simulink model "ctrl_typeA"  (R2016b)
settings: Solver=ode45  StartTime=0.0  StopTime=12.0  RelTol=1e-3  EnableMultiTasking=on
undefined symbols (not defined in the file): cMat_BF, cMat_IM, cMat_MN, cMat_TM, gain_actBFGAS, gain_actBFL, gain_actBFP, gain_actBFR, gain_actBFT, gain_actBFV, gain_actBFY, gain_actF0GAS, gain_actF1GAS, gain_actF2GAS, gain_actF3GAS, gain_actIML, gain_actIMP, gain_actIMR, gain_actIMT, gain_actIMV, gain_actIMY, gain_actIPL, gain_actIPT, gain_actIPY, gain_actMNL, gain_actMNP, gain_actMNR, gain_actMNT, gain_actMNV, gain_actMNY, gain_actTML, gain_actTMP, gain_actTMY, gainBFGAS, gainBFL, gainBFP, gainBFR, gainBFT, gainBFV, gainBFY, gainF0GAS, gainF1GAS, gainF2GAS, gainF3GAS, gainHieBFP, gainHieBFR, gainHieBFY, gainHieIML, gainHieIMP, gainHieIMY, gainHieIPL, gainHieIPY, gainHieMNL, gainHieMNP, gainHieMNY, gainIML, gainIMP, gainIMR, gainIMT, gainIMV ... (+24)
libraries: cstblocks x54
(part 2 of 2)

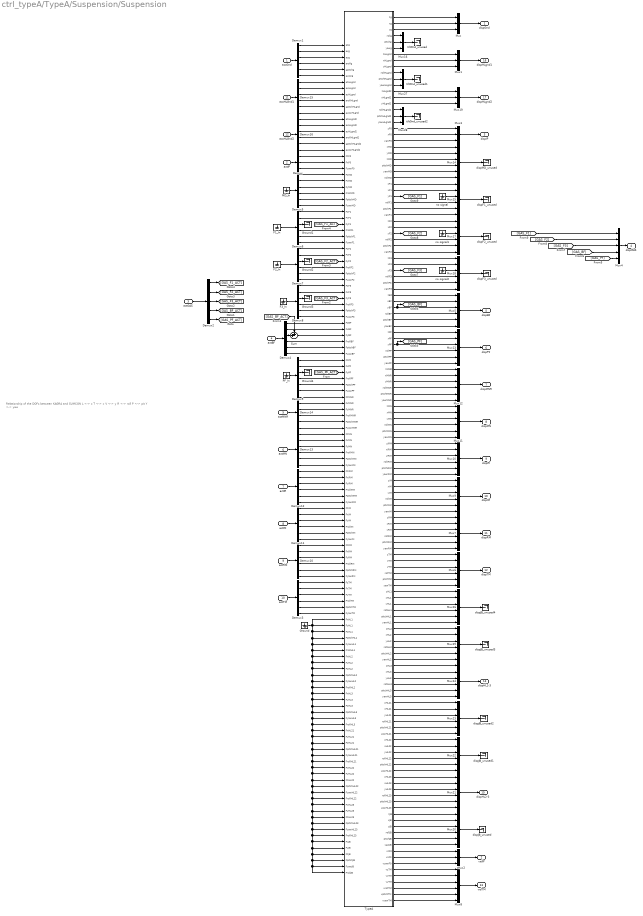
== system ctrl_typeA/TypeA/Suspension/Suspension ==
  note: Relationship of the DOFs
      | between KAGRA and SUMCON
      |
      | L <-> z
      | T <-> x
      | V <-> y
      | R <-> roll
      | P <-> pit
      | Y <-> yaw
  accGnd : Inport
  actIP : Inport  Port=2
  actGAS : Inport  Port=3
  actBF : Inport  Port=4
  actMNR : Inport  Port=5
  actMN : Inport  Port=6
  actIR : Inport  Port=7
  actIM : Inport  Port=8
  actRM : Inport  Port=9
  actTM : Inport  Port=10
  accHLGnd1 : Inport  Port=11
  accHLGnd2 : Inport  Port=12
  Demux : Demux  Outputs=3
  Demux{1,3..16} (15 alike) : Demux  Outputs=6
  Demux2 : Demux  Outputs=5
  F1_In : Ground
  F2_In : Ground
  F3_In : Ground
  Ground : Ground
  Ground{1..4} (4 alike) : Terminator
  MD_In : Ground
  Mux{,1..3,16,19,27..28} (8 alike) : Mux  Inputs=3
  Mux{5..15,17..18,20..26} (20 alike) : Mux  Inputs=6
  Mux4 : Mux  Inputs=5
  PF_In : Ground
  Sum : Sum  Inputs=++|
  TypeA : Subsystem
  dispF1_unused : Terminator
  dispF2_unused : Terminator
  dispF3_unused : Terminator
  dispJB_unused{,1..4} (5 alike) : Terminator
  dispMD_unused : Terminator
  no signal : Ground
  no signal1 : Ground
  no signal2 : Ground
  tiltGnd_unused : Terminator
  tiltGnd_unused1 : Terminator
  tiltGnd_unused2 : Terminator
  dispGnd : Outport
  velIP : Outport  Port=2
  dispIP : Outport  Port=3
  dispGAS : Outport  Port=4
  dispBF : Outport  Port=5
  dispPF : Outport  Port=6
  dispMNR : Outport  Port=7
  dispMN : Outport  Port=8
  dispIR : Outport  Port=9
  dispIM : Outport  Port=10
  dispRM : Outport  Port=11
  dispTM : Outport  Port=12
  velTM : Outport  Port=13
  dispHL1-3 : Outport  Port=14
  dispHL2-3 : Outport  Port=15
  dispHLgnd1 : Outport  Port=16
  dispHLgnd2 : Outport  Port=17
  wires:
  Mux/1 -> dispGnd/1
  Mux2/1 -> velIP/1
  Mux3/1 -> dispIP/1
  Mux4/1 -> dispGAS/1
  Mux5/1 -> dispBF/1
  Mux6/1 -> dispTM/1
  actIP/1 -> Demux/1
  accGnd/1 -> Demux1/1
  actTM/1 -> Demux3/1
  Demux4/3 -> Sum/2
  actBF/1 -> Demux4/1
  actGAS/1 -> Demux2/1
  MD_In/1 -> Demux5/1
  F1_In/1 -> Demux6/1
  F2_In/1 -> Demux7/1
  F3_In/1 -> Demux8/1
  Demux4/1 -> TypeA/46(FzBF)
  PF_In/1 -> Demux9/1
  actRM/1 -> Demux10/1
  actIM/1 -> Demux11/1
  actIR/1 -> Demux12/1
  actMN/1 -> Demux13/1
  actMNR/1 -> Demux14/1
  Demux10/5 -> TypeA/86(FpitchRM)
  Demux10/4 -> TypeA/85(FrollRM)
  Demux10/3 -> TypeA/84(FyRM)
  Demux10/1 -> TypeA/82(FzRM)
  Demux10/2 -> TypeA/83(FxRM)
  Demux3/3 -> TypeA/90(FyTM)
  Demux3/1 -> TypeA/88(FzTM)
  Demux3/2 -> TypeA/89(FxTM)
  Demux3/4 -> TypeA/91(FrollTM)
  Demux3/5 -> TypeA/92(FpitchTM)
  Demux3/6 -> TypeA/93(FyawTM)
  Mux7/1 -> dispRM/1
  Mux8/1 -> velTM/1
  Mux9/1 -> dispIM/1
  Mux10/1 -> dispIR/1
  Mux11/1 -> dispMN/1
  Mux12/1 -> dispMNR/1
  Mux13/1 -> dispPF/1
  Mux14/1 -> dispMD_unused/1
  Mux15/1 -> dispF1_unused/1
  Mux16/1 -> tiltGnd_unused/1
  Mux17/1 -> dispF2_unused/1
  Mux18/1 -> dispF3_unused/1
  TypeA/2(xg) -> Mux/2
  TypeA/1(zg) -> Mux/1
  TypeA/138(vyawF0) -> Mux2/3
  TypeA/20(xF0) -> Mux3/2
  TypeA/19(zF0) -> Mux3/1
  TypeA/21(yawF0) -> Mux3/3
  TypeA/24(zMD) -> Mux14/3
  TypeA/25(pitchMD) -> Mux14/4
  TypeA/26(yawMD) -> Mux14/5
  TypeA/27(rollMD) -> Mux14/6
  TypeA/48(yBF) -> Mux5/3, [GAS_BF]
  TypeA/54(yPF) -> [GAS_PF], Mux13/3
  TypeA/28(zF1) -> Mux15/1
  TypeA/29(xF1) -> Mux15/2
  TypeA/33(yawF1) -> Mux15/6
  TypeA/31(rollF1) -> Mux15/4
  TypeA/32(pitchF1) -> Mux15/5
  TypeA/34(zF2) -> Mux17/1
  TypeA/35(xF2) -> Mux17/2
  TypeA/37(rollF2) -> Mux17/4
  TypeA/39(yawF2) -> Mux17/6
  TypeA/38(pitchF2) -> Mux17/5
  TypeA/40(zF3) -> Mux18/1
  TypeA/41(xF3) -> Mux18/2
  TypeA/45(yawF3) -> Mux18/6
  TypeA/44(pitchF3) -> Mux18/5
  TypeA/43(rollF3) -> Mux18/4
  TypeA/50(pitchBF) -> Mux5/5
  TypeA/51(yawBF) -> Mux5/6
  TypeA/49(rollBF) -> Mux5/4
  TypeA/47(xBF) -> Mux5/2
  TypeA/46(zBF) -> Mux5/1
  TypeA/57(yawPF) -> Mux13/6
  TypeA/52(zPF) -> Mux13/1
  TypeA/53(xPF) -> Mux13/2
  TypeA/55(rollPF) -> Mux13/4
  TypeA/56(pitchPF) -> Mux13/5
  TypeA/59(xMNR) -> Mux12/2
  TypeA/63(yawMNR) -> Mux12/6
  TypeA/60(yMNR) -> Mux12/3
  TypeA/61(rollMNR) -> Mux12/4
  TypeA/58(zMNR) -> Mux12/1
  TypeA/62(pitchMNR) -> Mux12/5
  TypeA/67(rollMN) -> Mux11/4
  TypeA/64(zMN) -> Mux11/1
  TypeA/66(yMN) -> Mux11/3
  TypeA/65(xMN) -> Mux11/2
  TypeA/69(yawMN) -> Mux11/6
  TypeA/68(pitchMN) -> Mux11/5
  TypeA/74(pitchIRM) -> Mux10/5
  TypeA/72(yIRM) -> Mux10/3
  TypeA/75(yawIRM) -> Mux10/6
  TypeA/73(rollIRM) -> Mux10/4
  TypeA/71(xIRM) -> Mux10/2
  TypeA/70(zIRM) -> Mux10/1
  TypeA/76(zIM) -> Mux9/1
  TypeA/78(yIM) -> Mux9/3
  TypeA/77(xIM) -> Mux9/2
  TypeA/139(vzTM) -> Mux8/1
  TypeA/140(vxTM) -> Mux8/2
  TypeA/141(vyTM) -> Mux8/3
  TypeA/88(zTM) -> Mux6/1
  TypeA/89(xTM) -> Mux6/2
  TypeA/90(yTM) -> Mux6/3
  TypeA/82(zRM) -> Mux7/1
  TypeA/83(xRM) -> Mux7/2
  TypeA/84(yRM) -> Mux7/3
  TypeA/79(rollIM) -> Mux9/4
  TypeA/80(pitchIM) -> Mux9/5
  TypeA/81(yawIM) -> Mux9/6
  TypeA/85(rollRM) -> Mux7/4
  TypeA/86(pitchRM) -> Mux7/5
  TypeA/87(yawRM) -> Mux7/6
  TypeA/91(rollTM) -> Mux6/4
  TypeA/92(pitchTM) -> Mux6/5
  TypeA/93(yawTM) -> Mux6/6
  TypeA/22(xMD) -> Mux14/1
  TypeA/23(yMD) -> Mux14/2
  TypeA/137(vxF0) -> Mux2/2
  TypeA/136(vzF0) -> Mux2/1
  TypeA/3(yg) -> Mux/3
  Demux10/6 -> TypeA/87(FyawRM)
  Demux11/1 -> TypeA/76(FzIM)
  Demux11/2 -> TypeA/77(FxIM)
  Demux11/3 -> TypeA/78(FyIM)
  Demux11/4 -> TypeA/79(FrollIM)
  Demux11/5 -> TypeA/80(FpitchIM)
  Demux11/6 -> TypeA/81(FyawIM)
  Demux12/1 -> TypeA/70(FzIRM)
  Demux12/2 -> TypeA/71(FxIRM)
  Demux12/3 -> TypeA/72(FyIRM)
  Demux12/4 -> TypeA/73(FrollIRM)
  Demux12/5 -> TypeA/74(FpitchIRM)
  Demux12/6 -> TypeA/75(FyawIRM)
  Demux13/1 -> TypeA/64(FzMN)
  Demux13/2 -> TypeA/65(FxMN)
  Demux13/3 -> TypeA/66(FyMN)
  Demux13/4 -> TypeA/67(FrollMN)
  Demux13/5 -> TypeA/68(FpitchMN)
  Demux13/6 -> TypeA/69(FyawMN)
  Demux14/1 -> TypeA/58(FzMNR)
  Demux14/2 -> TypeA/59(FxMNR)
  Demux14/3 -> TypeA/60(FyMNR)
  Demux14/4 -> TypeA/61(FrollMNR)
  Demux14/5 -> TypeA/62(FpitchMNR)
  Demux14/6 -> TypeA/63(FyawMNR)
  Demux9/1 -> TypeA/52(FzPF)
  Demux9/2 -> TypeA/53(FxPF)
  Demux4/2 -> TypeA/47(FxBF)
  Sum/1 -> TypeA/48(FyBF)
  Demux4/4 -> TypeA/49(FrollBF)
  Demux4/5 -> TypeA/50(FpitchBF)
  Demux4/6 -> TypeA/51(FyawBF)
  Demux8/1 -> TypeA/40(FzF3)
  Demux8/2 -> TypeA/41(FxF3)
  Demux7/1 -> TypeA/34(FzF2)
  Demux7/2 -> TypeA/35(FxF2)
  Demux6/1 -> TypeA/28(FzF1)
  Demux6/2 -> TypeA/29(FxF1)
  Demux/1 -> TypeA/19(FzF0)
  Demux/2 -> TypeA/20(FxF0)
  Demux/3 -> TypeA/21(FyawF0)
  Demux1/1 -> TypeA/1(azg)
  Demux1/2 -> TypeA/2(axg)
  Demux1/3 -> TypeA/3(ayg)
  Demux1/4 -> TypeA/4(arollg)
  Demux1/5 -> TypeA/5(apitchg)
  Demux1/6 -> TypeA/6(ayawg)
  Mux20/1 -> dispJB_unused/1
  Mux21/1 -> dispHL2-3/1
  Mux22/1 -> dispJB_unused1/1
  Mux23/1 -> dispJB_unused2/1
  Mux24/1 -> dispHL1-3/1
  Mux25/1 -> dispJB_unused3/1
  Mux26/1 -> dispJB_unused4/1
  TypeA/7(zHLgnd) -> Mux1/1
  TypeA/8(xHLgnd) -> Mux1/2
  TypeA/9(yHLgnd) -> Mux1/3
  Mux1/1 -> dispHLgnd1/1
  Mux19/1 -> dispHLgnd2/1
  TypeA/15(yHLgnd2) -> Mux19/3
  TypeA/13(zHLgnd2) -> Mux19/1
  TypeA/14(xHLgnd2) -> Mux19/2
  Mux27/1 -> tiltGnd_unused1/1
  Mux28/1 -> tiltGnd_unused2/1
  Ground/1 -> TypeA/96(FzHL1), TypeA/97(FpitchHL1), TypeA/98(FyawHL1), TypeA/99(FrollHL1), TypeA/100(FxHL2), TypeA/101(FyHL2), TypeA/102(FzHL2), TypeA/103(FpitchHL2), TypeA/104(FyawHL2), TypeA/105(FrollHL2), TypeA/106(FxHL3), TypeA/107(FyHL3), TypeA/108(FzHL3), TypeA/109(FpitchHL3), TypeA/110(FyawHL3), TypeA/111(FrollHL3), TypeA/112(FxHL21), TypeA/113(FyHL21), TypeA/114(FzHL21), TypeA/115(FpitchHL21), TypeA/116(FyawHL21), TypeA/117(FrollHL21), TypeA/118(FxHL22), TypeA/119(FyHL22), TypeA/120(FzHL22), TypeA/121(FpitchHL22), TypeA/122(FyawHL22), TypeA/123(FrollHL22), TypeA/124(FxHL23), TypeA/125(FyHL23), TypeA/126(FzHL23), TypeA/127(FpitchHL23), TypeA/128(FyawHL23), TypeA/129(FrollHL23), TypeA/130(FxJB), TypeA/131(FyJB), TypeA/132(FzJB), TypeA/133(FpitchJB), TypeA/134(FyawJB), TypeA/135(FrollJB), TypeA/95(FyHL1), TypeA/94(FxHL1)
  Demux15/4 -> TypeA/10(arollHLgnd)
  Demux15/5 -> TypeA/11(apitchHLgnd)
  Demux15/1 -> TypeA/7(azHLgnd)
  Demux15/2 -> TypeA/8(axHLgnd)
  Demux15/6 -> TypeA/12(ayawHLgnd)
  accHLGnd1/1 -> Demux15/1
  Demux15/3 -> TypeA/9(ayHLgnd)
  Demux16/4 -> TypeA/16(arollHLgnd2)
  Demux16/5 -> TypeA/17(apitchHLgnd2)
  Demux16/1 -> TypeA/13(azHLgnd2)
  Demux16/2 -> TypeA/14(axHLgnd2)
  Demux16/6 -> TypeA/18(ayawHLgnd2)
  accHLGnd2/1 -> Demux16/1
  Demux16/3 -> TypeA/15(ayHLgnd2)
  Demux5/1 -> TypeA/22(FzMD)
  Demux5/2 -> TypeA/23(FxMD)
  Demux5/3 -> TypeA/24(FyMD)
  Demux5/4 -> TypeA/25(FrollMD)
  Demux5/5 -> TypeA/26(FpitchMD)
  Demux5/6 -> TypeA/27(FyawMD)
  Demux2/1 -> [GAS_F1_ACT]
  Demux2/2 -> [GAS_F2_ACT]
  Demux2/3 -> [GAS_F3_ACT]
  Demux2/4 -> [GAS_BF_ACT]
  Demux2/5 -> [GAS_PF_ACT]
  [GAS_F1_ACT] -> TypeA/30(FyF1)
  Demux6/4 -> TypeA/31(FrollF1)
  Demux6/3 -> Ground1/1
  Demux6/5 -> TypeA/32(FpitchF1)
  Demux6/6 -> TypeA/33(FyawF1)
  [GAS_F2_ACT] -> TypeA/36(FyF2)
  Demux7/5 -> TypeA/38(FpitchF2)
  Demux7/6 -> TypeA/39(FyawF2)
  Demux7/3 -> Ground2/1
  Demux7/4 -> TypeA/37(FrollF2)
  [GAS_F3_ACT] -> TypeA/42(FyF3)
  Demux8/3 -> Ground3/1
  Demux8/6 -> TypeA/45(FyawF3)
  Demux8/5 -> TypeA/44(FpitchF3)
  Demux8/4 -> TypeA/43(FrollF3)
  [GAS_BF_ACT] -> Sum/1
  [GAS_PF_ACT] -> TypeA/54(FyPF)
  Demux9/4 -> TypeA/55(FrollPF)
  Demux9/3 -> Ground4/1
  Demux9/5 -> TypeA/56(FpitchPF)
  Demux9/6 -> TypeA/57(FyawPF)
  TypeA/42(yF3) -> [GAS_F3]
  [GAS_PF] -> Mux4/5
  [GAS_BF] -> Mux4/4
  [GAS_F3] -> Mux4/3
  TypeA/36(yF2) -> [GAS_F2]
  TypeA/30(yF1) -> [GAS_F1]
  [GAS_F2] -> Mux4/2
  [GAS_F1] -> Mux4/1
  TypeA/4(rollg) -> Mux16/1
  TypeA/5(pitchg) -> Mux16/2
  TypeA/10(rollHLgnd) -> Mux27/1
  TypeA/11(pitchHLgnd) -> Mux27/2
  TypeA/16(rollHLgnd2) -> Mux28/1
  TypeA/17(pitchHLgnd2) -> Mux28/2
  no signal/1 -> Mux15/3
  no signal1/1 -> Mux17/3
  no signal2/1 -> Mux18/3
  TypeA/96(yHL1) -> Mux26/3
  TypeA/95(xHL1) -> Mux26/2
  TypeA/94(zHL1) -> Mux26/1
  TypeA/99(yawHL1) -> Mux26/6
  TypeA/98(pitchHL1) -> Mux26/5
  TypeA/97(rollHL1) -> Mux26/4
  TypeA/100(zHL2) -> Mux25/1
  TypeA/101(xHL2) -> Mux25/2
  TypeA/102(yHL2) -> Mux25/3
  TypeA/103(rollHL2) -> Mux25/4
  TypeA/104(pitchHL2) -> Mux25/5
  TypeA/105(yawHL2) -> Mux25/6
  TypeA/107(xHL3) -> Mux24/2
  TypeA/108(yHL3) -> Mux24/3
  TypeA/109(rollHL3) -> Mux24/4
  TypeA/110(pitchHL3) -> Mux24/5
  TypeA/111(yawHL3) -> Mux24/6
  TypeA/106(zHL3) -> Mux24/1
  TypeA/112(zHL21) -> Mux23/1
  TypeA/113(xHL21) -> Mux23/2
  TypeA/114(yHL21) -> Mux23/3
  TypeA/115(rollHL21) -> Mux23/4
  TypeA/116(pitchHL21) -> Mux23/5
  TypeA/117(yawHL21) -> Mux23/6
  TypeA/119(xHL22) -> Mux22/2
  TypeA/120(yHL22) -> Mux22/3
  TypeA/118(zHL22) -> Mux22/1
  TypeA/122(pitchHL22) -> Mux22/5
  TypeA/123(yawHL22) -> Mux22/6
  TypeA/121(rollHL22) -> Mux22/4
  TypeA/125(xHL23) -> Mux21/2
  TypeA/126(yHL23) -> Mux21/3
  TypeA/124(zHL23) -> Mux21/1
  TypeA/128(pitchHL23) -> Mux21/5
  TypeA/129(yawHL23) -> Mux21/6
  TypeA/127(rollHL23) -> Mux21/4
  TypeA/131(xJB) -> Mux20/2
  TypeA/132(yJB) -> Mux20/3
  TypeA/130(zJB) -> Mux20/1
  TypeA/134(pitchJB) -> Mux20/5
  TypeA/135(yawJB) -> Mux20/6
  TypeA/133(rollJB) -> Mux20/4
  TypeA/143(vpitchTM) -> Mux8/5
  TypeA/144(vyawTM) -> Mux8/6
  TypeA/142(vrollTM) -> Mux8/4
  TypeA/6(yawg) -> Mux16/3
  TypeA/12(yawHLgnd) -> Mux27/3
  TypeA/18(yawHLgnd2) -> Mux28/3

== system ctrl_typeA/TypeA/Suspension/aMatrix_BF ==
  aMat_in : Inport
  cMat_BF : Constant  Value=cMat_BF  VectorParams1D=off
  coupling_BF : Product  Multiplication=Matrix(*)
  actBF : Outport
  wires:
  coupling_BF/1 -> actBF/1
  aMat_in/1 -> coupling_BF/2
  cMat_BF/1 -> coupling_BF/1

== system ctrl_typeA/TypeA/Suspension/aMatrix_GAS ==
  aMat_in : Inport
  Add{1..4} (4 alike) : Sum  Inputs=+-
  Demux4 : Demux  Outputs=5
  Mux3 : Mux  Inputs=5
  actGAS : Outport
  wires:
  aMat_in/1 -> Demux4/1
  Mux3/1 -> actGAS/1
  Add1/1 -> Mux3/1
  Add2/1 -> Mux3/2
  Demux4/3 -> Add3/1, Add2/2
  Demux4/2 -> Add1/2, Add2/1
  Demux4/1 -> Add1/1
  Demux4/5 -> Mux3/5, Add4/2
  Add4/1 -> Mux3/4
  Add3/1 -> Mux3/3
  Demux4/4 -> Add3/2, Add4/1

== system ctrl_typeA/TypeA/Suspension/aMatrix_IM ==
  aMat_in : Inport
  Gain : Gain  Gain=-1
  cMat_IM : Constant  Value=cMat_IM  VectorParams1D=off
  coupling_IM : Product  Multiplication=Matrix(*)
  actIR : Outport
  actIM : Outport  Port=2
  wires:
  coupling_IM/1 -> actIM/1, Gain/1
  aMat_in/1 -> coupling_IM/2
  cMat_IM/1 -> coupling_IM/1
  Gain/1 -> actIR/1

== system ctrl_typeA/TypeA/Suspension/aMatrix_MN ==
  aMat_in : Inport
  Gain : Gain  Gain=-1
  cMat_MN : Constant  Value=cMat_MN  VectorParams1D=off
  coupling_MN : Product  Multiplication=Matrix(*)
  actMNR : Outport
  actMN : Outport  Port=2
  wires:
  coupling_MN/1 -> actMN/1, Gain/1
  aMat_in/1 -> coupling_MN/2
  cMat_MN/1 -> coupling_MN/1
  Gain/1 -> actMNR/1

== system ctrl_typeA/TypeA/Suspension/aMatrix_TM ==
  aMat_in : Inport
  Demux : Demux  Outputs=3
  Demux1 : Demux  Outputs=3
  Gain : Gain  Gain=-1
  Ground{,1..5} (6 alike) : Ground
  Mux : Mux  Inputs=6
  Mux1 : Mux  Inputs=6
  cMat_TM : Constant  Value=cMat_TM  VectorParams1D=off
  coupling_TM : Product  Multiplication=Matrix(*)
  actRM : Outport
  actTM : Outport  Port=2
  wires:
  coupling_TM/1 -> Demux1/1, Gain/1
  aMat_in/1 -> coupling_TM/2  "3DoF"
  cMat_TM/1 -> coupling_TM/1
  Gain/1 -> Demux/1
  Demux/1 -> Mux/1
  Demux/2 -> Mux/5
  Demux/3 -> Mux/6
  Demux1/1 -> Mux1/1
  Demux1/3 -> Mux1/6
  Demux1/2 -> Mux1/5
  Ground/1 -> Mux/2
  Ground1/1 -> Mux/3
  Ground2/1 -> Mux/4
  Ground4/1 -> Mux1/3
  Ground3/1 -> Mux1/2
  Ground5/1 -> Mux1/4
  Mux/1 -> actRM/1  "6DoF"
  Mux1/1 -> actTM/1  "6DoF"

== system ctrl_typeA/TypeA/Suspension/sMatrix_BF_LVDT ==
  dispGnd : Inport
  dispBF : Inport  Port=2
  Add2 : Sum  Inputs=-+
  Demux : Demux  Outputs=3
  Ground : Ground
  Ground1 : Ground
  Ground2 : Ground
  Mux : Mux  Inputs=6
  BF_LVDT : Outport
  wires:
  Add2/1 -> BF_LVDT/1  "6DoF"
  dispBF/1 -> Add2/2  "6DoF"
  dispGnd/1 -> Demux/1  "3DoF"
  Demux/1 -> Mux/1  "L"
  Demux/2 -> Mux/2  "T"
  Demux/3 -> Mux/3  "V"
  Ground/1 -> Mux/4  "R"
  Ground1/1 -> Mux/5  "P"
  Mux/1 -> Add2/1
  Ground2/1 -> Mux/6  "Y"

== system ctrl_typeA/TypeA/Suspension/sMatrix_GAS_LVDT ==
  dispGAS : Inport
  dispGND : Inport  Port=2
  Add{1..5} (5 alike) : Sum  Inputs=-+
  Demux : Demux  Outputs=3
  Demux4 : Demux  Outputs=5
  Mux3 : Mux  Inputs=5
  Terminator1 : Terminator
  Terminator2 : Terminator
  GAS_LVDT : Outport
  wires:
  dispGAS/1 -> Demux4/1
  Demux4/1 -> Add2/2, Add1/1  "VF1"
  Demux4/2 -> Add3/1, Add1/2  "VF2"
  Demux4/3 -> Add4/1, Add3/2  "VF3"
  Add2/1 -> Mux3/1  "GASF0"
  Add1/1 -> Mux3/2  "GASF1"
  Add3/1 -> Mux3/3  "GASF2"
  Mux3/1 -> GAS_LVDT/1
  Demux4/4 -> Add5/1, Add4/2  "VBF"
  Demux4/5 -> Add5/2  "VPF"
  Add4/1 -> Mux3/4  "GASF3"
  Add5/1 -> Mux3/5  "GASBF"
  dispGND/1 -> Demux/1
  Demux/3 -> Add2/1  "GND_V"
  Demux/2 -> Terminator1/1  "T"
  Demux/1 -> Terminator2/1  "L"

== system ctrl_typeA/TypeA/Suspension/sMatrix_IM_OpLev ==
  dispIM : Inport
  dispGND : Inport  Port=2
  Add2 : Sum  Inputs=-+
  Demux1 : Demux  Outputs=3
  Demux4 : Demux  Outputs=6
  Mux1 : Mux  Inputs=3
  Mux3 : Mux  Inputs=3
  dispGNDP1 : Ground
  dispGNDT : Terminator
  dispGNDV : Terminator
  dispGNDY1 : Ground
  dispTMR : Terminator
  dispTMT : Terminator
  dispTMV : Terminator
  IM_OpLev : Outport
  wires:
  dispIM/1 -> Demux4/1
  Mux3/1 -> Add2/1
  Demux4/1 -> Mux3/1  "L"
  Demux4/2 -> dispTMT/1
  Demux4/3 -> dispTMV/1
  Demux4/4 -> dispTMR/1
  Demux4/5 -> Mux3/2  "P"
  Demux4/6 -> Mux3/3  "Y"
  Demux1/1 -> Mux1/1  "L"
  Demux1/2 -> dispGNDT/1
  Demux1/3 -> dispGNDV/1
  dispGND/1 -> Demux1/1
  dispGNDP1/1 -> Mux1/2  "P"
  Mux1/1 -> Add2/2
  Add2/1 -> IM_OpLev/1
  dispGNDY1/1 -> Mux1/3  "Y"

== system ctrl_typeA/TypeA/Suspension/sMatrix_IM_PS ==
  dispIR : Inport
  dispIM : Inport  Port=2
  Add2 : Sum  Inputs=-+
  IM_PS : Outport
  wires:
  Add2/1 -> IM_PS/1
  dispIM/1 -> Add2/2
  dispIR/1 -> Add2/1

== system ctrl_typeA/TypeA/Suspension/sMatrix_IP_LVDT ==
  dispGnd : Inport
  dispIP : Inport  Port=2
  Add2 : Sum  Inputs=-+
  Demux : Demux  Outputs=3
  Mux : Mux  Inputs=3
  Terminator : Terminator
  no signal : Ground
  IP_LVDT : Outport
  wires:
  Add2/1 -> IP_LVDT/1
  dispIP/1 -> Add2/2  "L,T,Y"
  dispGnd/1 -> Demux/1
  Demux/1 -> Mux/1  "L"
  Demux/2 -> Mux/2  "T"
  Demux/3 -> Terminator/1  "V"
  Mux/1 -> Add2/1
  no signal/1 -> Mux/3  "Y"

== system ctrl_typeA/TypeA/Suspension/sMatrix_MN_OpLev ==
  dispMN : Inport
  dispGND : Inport  Port=2
  Add2 : Sum  Inputs=-+
  Demux1 : Demux  Outputs=3
  Demux4 : Demux  Outputs=6
  Mux1 : Mux  Inputs=3
  Mux3 : Mux  Inputs=3
  dispGNDP1 : Ground
  dispGNDT : Terminator
  dispGNDV : Terminator
  dispGNDY1 : Ground
  dispTMR : Terminator
  dispTMT : Terminator
  dispTMV : Terminator
  MN_OpLev : Outport
  wires:
  dispMN/1 -> Demux4/1
  Mux3/1 -> Add2/1
  Demux4/1 -> Mux3/1  "L"
  Demux4/2 -> dispTMT/1
  Demux4/3 -> dispTMV/1
  Demux4/4 -> dispTMR/1
  Demux4/5 -> Mux3/2  "P"
  Demux4/6 -> Mux3/3  "Y"
  Demux1/1 -> Mux1/1  "L"
  Demux1/2 -> dispGNDT/1
  Demux1/3 -> dispGNDV/1
  dispGND/1 -> Demux1/1
  dispGNDP1/1 -> Mux1/2  "P"
  Mux1/1 -> Add2/2
  Add2/1 -> MN_OpLev/1
  dispGNDY1/1 -> Mux1/3  "Y"

== system ctrl_typeA/TypeA/Suspension/sMatrix_MN_PS ==
  dispMNR : Inport
  dispMN : Inport  Port=2
  Add2 : Sum  Inputs=-+
  MN_PS : Outport
  wires:
  Add2/1 -> MN_PS/1
  dispMN/1 -> Add2/2
  dispMNR/1 -> Add2/1

== system ctrl_typeA/TypeA/Suspension/sMatrix_PF_OpLev ==
  dispPF : Inport
  dispGND : Inport  Port=2
  Add2 : Sum  Inputs=-+
  Demux1 : Demux  Outputs=3
  Demux4 : Demux  Outputs=6
  Mux1 : Mux  Inputs=3
  Mux3 : Mux  Inputs=3
  dispGNDP1 : Ground
  dispGNDT : Terminator
  dispGNDV : Terminator
  dispGNDY1 : Ground
  dispTMR : Terminator
  dispTMT : Terminator
  dispTMV : Terminator
  PF_OpLev : Outport
  wires:
  dispPF/1 -> Demux4/1
  Mux3/1 -> Add2/1
  Demux4/1 -> Mux3/1  "L"
  Demux4/2 -> dispTMT/1
  Demux4/3 -> dispTMV/1
  Demux4/4 -> dispTMR/1
  Demux4/5 -> Mux3/2  "P"
  Demux4/6 -> Mux3/3  "Y"
  Demux1/1 -> Mux1/1  "L"
  Demux1/2 -> dispGNDT/1
  Demux1/3 -> dispGNDV/1
  dispGND/1 -> Demux1/1
  dispGNDP1/1 -> Mux1/2  "P"
  Mux1/1 -> Add2/2
  Add2/1 -> PF_OpLev/1
  dispGNDY1/1 -> Mux1/3  "Y"

== system ctrl_typeA/TypeA/Suspension/sMatrix_TM_OpLev ==
  dispTM : Inport
  dispGND : Inport  Port=2
  Add2 : Sum  Inputs=-+
  Demux1 : Demux  Outputs=3
  Demux4 : Demux  Outputs=6
  Mux1 : Mux  Inputs=3
  Mux3 : Mux  Inputs=3
  dispGNDP1 : Ground
  dispGNDT : Terminator
  dispGNDV : Terminator
  dispGNDY1 : Ground
  dispTMR : Terminator
  dispTMT : Terminator
  dispTMV : Terminator
  TM_OpLev : Outport
  wires:
  dispTM/1 -> Demux4/1
  Mux3/1 -> Add2/1
  Demux4/1 -> Mux3/1  "L"
  Demux4/2 -> dispTMT/1
  Demux4/3 -> dispTMV/1
  Demux4/4 -> dispTMR/1
  Demux4/5 -> Mux3/2  "P"
  Demux4/6 -> Mux3/3  "Y"
  Demux1/1 -> Mux1/1  "L"
  Demux1/2 -> dispGNDT/1
  Demux1/3 -> dispGNDV/1
  dispGND/1 -> Demux1/1
  dispGNDP1/1 -> Mux1/2  "P"
  Mux1/1 -> Add2/2
  Add2/1 -> TM_OpLev/1
  dispGNDY1/1 -> Mux1/3  "Y"

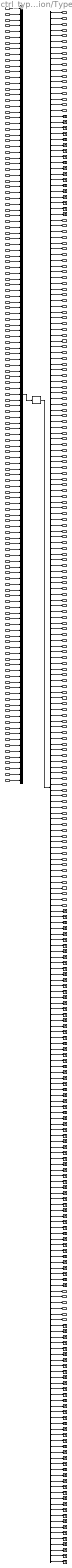
== system ctrl_typeA/TypeA/Suspension/Suspension/TypeA ==
  azg : Inport
  axg : Inport  Port=2
  ayg : Inport  Port=3
  arollg : Inport  Port=4
  apitchg : Inport  Port=5
  ayawg : Inport  Port=6
  azHLgnd : Inport  Port=7
  axHLgnd : Inport  Port=8
  ayHLgnd : Inport  Port=9
  arollHLgnd : Inport  Port=10
  apitchHLgnd : Inport  Port=11
  ayawHLgnd : Inport  Port=12
  azHLgnd2 : Inport  Port=13
  axHLgnd2 : Inport  Port=14
  ayHLgnd2 : Inport  Port=15
  arollHLgnd2 : Inport  Port=16
  apitchHLgnd2 : Inport  Port=17
  ayawHLgnd2 : Inport  Port=18
  FzF0 : Inport  Port=19
  FxF0 : Inport  Port=20
  FyawF0 : Inport  Port=21
  FzMD : Inport  Port=22
  FxMD : Inport  Port=23
  FyMD : Inport  Port=24
  FrollMD : Inport  Port=25
  FpitchMD : Inport  Port=26
  FyawMD : Inport  Port=27
  FzF1 : Inport  Port=28
  FxF1 : Inport  Port=29
  FyF1 : Inport  Port=30
  FrollF1 : Inport  Port=31
  FpitchF1 : Inport  Port=32
  FyawF1 : Inport  Port=33
  FzF2 : Inport  Port=34
  FxF2 : Inport  Port=35
  FyF2 : Inport  Port=36
  FrollF2 : Inport  Port=37
  FpitchF2 : Inport  Port=38
  FyawF2 : Inport  Port=39
  FzF3 : Inport  Port=40
  FxF3 : Inport  Port=41
  FyF3 : Inport  Port=42
  FrollF3 : Inport  Port=43
  FpitchF3 : Inport  Port=44
  FyawF3 : Inport  Port=45
  FzBF : Inport  Port=46
  FxBF : Inport  Port=47
  FyBF : Inport  Port=48
  FrollBF : Inport  Port=49
  FpitchBF : Inport  Port=50
  FyawBF : Inport  Port=51
  FzPF : Inport  Port=52
  FxPF : Inport  Port=53
  FyPF : Inport  Port=54
  FrollPF : Inport  Port=55
  FpitchPF : Inport  Port=56
  FyawPF : Inport  Port=57
  FzMNR : Inport  Port=58
  FxMNR : Inport  Port=59
  FyMNR : Inport  Port=60
  FrollMNR : Inport  Port=61
  FpitchMNR : Inport  Port=62
  FyawMNR : Inport  Port=63
  FzMN : Inport  Port=64
  FxMN : Inport  Port=65
  FyMN : Inport  Port=66
  FrollMN : Inport  Port=67
  FpitchMN : Inport  Port=68
  FyawMN : Inport  Port=69
  FzIRM : Inport  Port=70
  FxIRM : Inport  Port=71
  FyIRM : Inport  Port=72
  FrollIRM : Inport  Port=73
  FpitchIRM : Inport  Port=74
  FyawIRM : Inport  Port=75
  FzIM : Inport  Port=76
  FxIM : Inport  Port=77
  FyIM : Inport  Port=78
  FrollIM : Inport  Port=79
  FpitchIM : Inport  Port=80
  FyawIM : Inport  Port=81
  FzRM : Inport  Port=82
  FxRM : Inport  Port=83
  FyRM : Inport  Port=84
  FrollRM : Inport  Port=85
  FpitchRM : Inport  Port=86
  FyawRM : Inport  Port=87
  FzTM : Inport  Port=88
  FxTM : Inport  Port=89
  FyTM : Inport  Port=90
  FrollTM : Inport  Port=91
  FpitchTM : Inport  Port=92
  FyawTM : Inport  Port=93
  FxHL1 : Inport  Port=94
  FyHL1 : Inport  Port=95
  FzHL1 : Inport  Port=96
  FpitchHL1 : Inport  Port=97
  FyawHL1 : Inport  Port=98
  FrollHL1 : Inport  Port=99
  FxHL2 : Inport  Port=100
  FyHL2 : Inport  Port=101
  FzHL2 : Inport  Port=102
  FpitchHL2 : Inport  Port=103
  FyawHL2 : Inport  Port=104
  FrollHL2 : Inport  Port=105
  FxHL3 : Inport  Port=106
  FyHL3 : Inport  Port=107
  FzHL3 : Inport  Port=108
  FpitchHL3 : Inport  Port=109
  FyawHL3 : Inport  Port=110
  FrollHL3 : Inport  Port=111
  FxHL21 : Inport  Port=112
  FyHL21 : Inport  Port=113
  FzHL21 : Inport  Port=114
  FpitchHL21 : Inport  Port=115
  FyawHL21 : Inport  Port=116
  FrollHL21 : Inport  Port=117
  FxHL22 : Inport  Port=118
  FyHL22 : Inport  Port=119
  FzHL22 : Inport  Port=120
  FpitchHL22 : Inport  Port=121
  FyawHL22 : Inport  Port=122
  FrollHL22 : Inport  Port=123
  FxHL23 : Inport  Port=124
  FyHL23 : Inport  Port=125
  FzHL23 : Inport  Port=126
  FpitchHL23 : Inport  Port=127
  FyawHL23 : Inport  Port=128
  FrollHL23 : Inport  Port=129
  FxJB : Inport  Port=130
  FyJB : Inport  Port=131
  FzJB : Inport  Port=132
  FpitchJB : Inport  Port=133
  FyawJB : Inport  Port=134
  FrollJB : Inport  Port=135
  SAS State-Space : StateSpace  A=ssA  B=ssB  C=ssC  D=ssD  X0=0  ContinuousStateAttributes='SUS_SS_MODEL'
  Terminator{,1..125} (126 alike) : Terminator
  demux : Demux  Outputs=270
  mux : Mux  Inputs=135
  zg : Outport
  xg : Outport  Port=2
  yg : Outport  Port=3
  rollg : Outport  Port=4
  pitchg : Outport  Port=5
  yawg : Outport  Port=6
  zHLgnd : Outport  Port=7
  xHLgnd : Outport  Port=8
  yHLgnd : Outport  Port=9
  rollHLgnd : Outport  Port=10
  pitchHLgnd : Outport  Port=11
  yawHLgnd : Outport  Port=12
  zHLgnd2 : Outport  Port=13
  xHLgnd2 : Outport  Port=14
  yHLgnd2 : Outport  Port=15
  rollHLgnd2 : Outport  Port=16
  pitchHLgnd2 : Outport  Port=17
  yawHLgnd2 : Outport  Port=18
  zF0 : Outport  Port=19
  xF0 : Outport  Port=20
  yawF0 : Outport  Port=21
  xMD : Outport  Port=22
  yMD : Outport  Port=23
  zMD : Outport  Port=24
  pitchMD : Outport  Port=25
  yawMD : Outport  Port=26
  rollMD : Outport  Port=27
  zF1 : Outport  Port=28
  xF1 : Outport  Port=29
  yF1 : Outport  Port=30
  rollF1 : Outport  Port=31
  pitchF1 : Outport  Port=32
  yawF1 : Outport  Port=33
  zF2 : Outport  Port=34
  xF2 : Outport  Port=35
  yF2 : Outport  Port=36
  rollF2 : Outport  Port=37
  pitchF2 : Outport  Port=38
  yawF2 : Outport  Port=39
  zF3 : Outport  Port=40
  xF3 : Outport  Port=41
  yF3 : Outport  Port=42
  rollF3 : Outport  Port=43
  pitchF3 : Outport  Port=44
  yawF3 : Outport  Port=45
  zBF : Outport  Port=46
  xBF : Outport  Port=47
  yBF : Outport  Port=48
  rollBF : Outport  Port=49
  pitchBF : Outport  Port=50
  yawBF : Outport  Port=51
  zPF : Outport  Port=52
  xPF : Outport  Port=53
  yPF : Outport  Port=54
  rollPF : Outport  Port=55
  pitchPF : Outport  Port=56
  yawPF : Outport  Port=57
  zMNR : Outport  Port=58
  xMNR : Outport  Port=59
  yMNR : Outport  Port=60
  rollMNR : Outport  Port=61
  pitchMNR : Outport  Port=62
  yawMNR : Outport  Port=63
  zMN : Outport  Port=64
  xMN : Outport  Port=65
  yMN : Outport  Port=66
  rollMN : Outport  Port=67
  pitchMN : Outport  Port=68
  yawMN : Outport  Port=69
  zIRM : Outport  Port=70
  xIRM : Outport  Port=71
  yIRM : Outport  Port=72
  rollIRM : Outport  Port=73
  pitchIRM : Outport  Port=74
  yawIRM : Outport  Port=75
  zIM : Outport  Port=76
  xIM : Outport  Port=77
  yIM : Outport  Port=78
  rollIM : Outport  Port=79
  pitchIM : Outport  Port=80
  yawIM : Outport  Port=81
  zRM : Outport  Port=82
  xRM : Outport  Port=83
  yRM : Outport  Port=84
  rollRM : Outport  Port=85
  pitchRM : Outport  Port=86
  yawRM : Outport  Port=87
  zTM : Outport  Port=88
  xTM : Outport  Port=89
  yTM : Outport  Port=90
  rollTM : Outport  Port=91
  pitchTM : Outport  Port=92
  yawTM : Outport  Port=93
  zHL1 : Outport  Port=94
  xHL1 : Outport  Port=95
  yHL1 : Outport  Port=96
  rollHL1 : Outport  Port=97
  pitchHL1 : Outport  Port=98
  yawHL1 : Outport  Port=99
  zHL2 : Outport  Port=100
  xHL2 : Outport  Port=101
  yHL2 : Outport  Port=102
  rollHL2 : Outport  Port=103
  pitchHL2 : Outport  Port=104
  yawHL2 : Outport  Port=105
  zHL3 : Outport  Port=106
  xHL3 : Outport  Port=107
  yHL3 : Outport  Port=108
  rollHL3 : Outport  Port=109
  pitchHL3 : Outport  Port=110
  yawHL3 : Outport  Port=111
  zHL21 : Outport  Port=112
  xHL21 : Outport  Port=113
  yHL21 : Outport  Port=114
  rollHL21 : Outport  Port=115
  pitchHL21 : Outport  Port=116
  yawHL21 : Outport  Port=117
  zHL22 : Outport  Port=118
  xHL22 : Outport  Port=119
  yHL22 : Outport  Port=120
  rollHL22 : Outport  Port=121
  pitchHL22 : Outport  Port=122
  yawHL22 : Outport  Port=123
  zHL23 : Outport  Port=124
  xHL23 : Outport  Port=125
  yHL23 : Outport  Port=126
  rollHL23 : Outport  Port=127
  pitchHL23 : Outport  Port=128
  yawHL23 : Outport  Port=129
  zJB : Outport  Port=130
  xJB : Outport  Port=131
  yJB : Outport  Port=132
  rollJB : Outport  Port=133
  pitchJB : Outport  Port=134
  yawJB : Outport  Port=135
  vzF0 : Outport  Port=136
  vxF0 : Outport  Port=137
  vyawF0 : Outport  Port=138
  vzTM : Outport  Port=139
  vxTM : Outport  Port=140
  vyTM : Outport  Port=141
  vrollTM : Outport  Port=142
  vpitchTM : Outport  Port=143
  vyawTM : Outport  Port=144
  wires:
  demux/165 -> Terminator26/1
  demux/265 -> Terminator120/1
  demux/247 -> Terminator102/1
  demux/191 -> Terminator52/1
  FrollHL23/1 -> mux/129
  demux/163 -> Terminator24/1
  FzIM/1 -> mux/78
  demux/263 -> Terminator118/1
  demux/260 -> Terminator115/1
  SAS State-Space/1 -> demux/1
  arollHLgnd2/1 -> mux/18
  demux/236 -> Terminator91/1
  demux/256 -> Terminator111/1
  demux/183 -> Terminator44/1
  demux/255 -> Terminator110/1
  demux/242 -> Terminator97/1
  demux/252 -> Terminator107/1
  demux/137 -> yHL22/1
  demux/75 -> rollPF/1
  demux/234 -> Terminator89/1
  FzF1/1 -> mux/30
  demux/177 -> Terminator38/1
  FzF3/1 -> mux/42
  demux/251 -> Terminator106/1
  demux/243 -> Terminator98/1
  demux/227 -> vyawTM/1
  demux/173 -> Terminator34/1
  demux/78 -> zMNR/1
  demux/106 -> xTM/1
  demux/228 -> vrollTM/1
  demux/246 -> Terminator101/1
  demux/120 -> zHL2/1
  demux/223 -> vxTM/1
  demux/239 -> Terminator94/1
  demux/241 -> Terminator96/1
  demux/216 -> Terminator77/1
  demux/215 -> Terminator76/1
  demux/107 -> yTM/1
  demux/206 -> Terminator67/1
  demux/235 -> Terminator90/1
  demux/237 -> Terminator92/1
  demux/203 -> Terminator64/1
  demux/233 -> Terminator88/1
  demux/224 -> vyTM/1
  demux/155 -> vzF0/1
  demux/266 -> Terminator121/1
  demux/238 -> Terminator93/1
  demux/270 -> Terminator125/1
  demux/232 -> Terminator87/1
  demux/244 -> Terminator99/1
  FzIRM/1 -> mux/72
  demux/248 -> Terminator103/1
  FyF3/1 -> mux/41
  demux/253 -> Terminator108/1
  demux/249 -> Terminator104/1
  demux/122 -> yawHL2/1
  demux/175 -> Terminator36/1
  demux/202 -> Terminator63/1
  demux/268 -> Terminator123/1
  demux/164 -> Terminator25/1
  demux/218 -> Terminator79/1
  FzHL1/1 -> mux/96
  demux/261 -> Terminator116/1
  demux/254 -> Terminator109/1
  demux/269 -> Terminator124/1
  demux/174 -> Terminator35/1
  demux/57 -> rollF2/1
  demux/171 -> Terminator32/1
  FyBF/1 -> mux/47
  FyawIM/1 -> mux/80
  demux/176 -> Terminator37/1
  FpitchMNR/1 -> mux/61
  demux/140 -> yawHL22/1
  demux/149 -> yJB/1
  demux/146 -> yawHL23/1
  demux/226 -> vpitchTM/1
  demux/162 -> Terminator23/1
  FxMNR/1 -> mux/58
  demux/74 -> yawPF/1
  demux/56 -> yawF2/1
  demux/153 -> rollJB/1
  demux/219 -> Terminator80/1
  FrollTM/1 -> mux/93
  demux/142 -> xHL23/1
  demux/240 -> Terminator95/1
  demux/159 -> Terminator20/1
  demux/145 -> pitchHL23/1
  demux/130 -> xHL21/1
  demux/204 -> Terminator65/1
  demux/129 -> rollHL3/1
  demux/128 -> yawHL3/1
  FpitchMD/1 -> mux/25
  demux/135 -> rollHL21/1
  axg/1 -> mux/1
  demux/267 -> Terminator122/1
  demux/139 -> pitchHL22/1
  demux/136 -> xHL22/1
  demux/222 -> Terminator83/1
  demux/131 -> yHL21/1
  demux/73 -> pitchPF/1
  demux/121 -> pitchHL2/1
  demux/104 -> yawRM/1
  apitchg/1 -> mux/4
  demux/250 -> Terminator105/1
  demux/124 -> xHL3/1
  demux/113 -> yHL1/1
  demux/117 -> rollHL1/1
  demux/63 -> rollF3/1
  demux/109 -> pitchTM/1
  demux/126 -> zHL3/1
  demux/198 -> Terminator59/1
  demux/96 -> zIM/1
  FzMD/1 -> mux/24
  demux/264 -> Terminator119/1
  FrollMD/1 -> mux/27
  FzHL21/1 -> mux/114
  demux/112 -> xHL1/1
  demux/144 -> zHL23/1
  FxF1/1 -> mux/28
  demux/108 -> zTM/1
  demux/213 -> Terminator74/1
  demux/102 -> zRM/1
  FyawF1/1 -> mux/32
  demux/211 -> Terminator72/1
  demux/94 -> xIM/1
  demux/41 -> yMD/1
  demux/101 -> yRM/1
  demux/158 -> Terminator19/1
  demux/103 -> pitchRM/1
  demux/152 -> yawJB/1
  demux/231 -> Terminator86/1
  demux/15 -> zHLgnd2/1
  demux/46 -> xF1/1
  demux/127 -> pitchHL3/1
  demux/38 -> zF0/1
  FxMD/1 -> mux/22
  demux/86 -> yawMN/1
  demux/91 -> pitchIRM/1
  FyawRM/1 -> mux/86
  demux/262 -> Terminator117/1
  demux/89 -> yIRM/1
  demux/8 -> yHLgnd/1
  demux/81 -> rollMNR/1
  demux/123 -> rollHL2/1
  demux/19 -> Terminator/1
  demux/168 -> Terminator29/1
  demux/77 -> yMNR/1
  demux/80 -> yawMNR/1
  demux/79 -> pitchMNR/1
  demux/58 -> xF3/1
  demux/82 -> xMN/1
  demux/210 -> Terminator71/1
  demux/68 -> yawBF/1
  demux/54 -> zF2/1
  demux/26 -> Terminator7/1
  demux/66 -> zBF/1
  demux/64 -> xBF/1
  demux/125 -> yHL3/1
  FyRM/1 -> mux/83
  FyPF/1 -> mux/53
  demux/53 -> yF2/1
  FyHL1/1 -> mux/95
  demux/225 -> vzTM/1
  demux/60 -> zF3/1
  demux/220 -> Terminator81/1
  demux/199 -> Terminator60/1
  FxF0/1 -> mux/19
  FzF2/1 -> mux/36
  demux/52 -> xF2/1
  FrollHL3/1 -> mux/111
  demux/43 -> pitchMD/1
  demux/22 -> Terminator3/1
  demux/92 -> yawIRM/1
  demux/150 -> zJB/1
  demux/13 -> xHLgnd2/1
  demux/40 -> xMD/1
  demux/50 -> yawF1/1
  demux/49 -> pitchF1/1
  demux/118 -> xHL2/1
  demux/99 -> rollIM/1
  demux/44 -> yawMD/1
  demux/48 -> zF1/1
  demux/134 -> yawHL21/1
  FxPF/1 -> mux/52
  demux/28 -> Terminator9/1
  demux/62 -> yawF3/1
  demux/132 -> zHL21/1
  demux/4 -> pitchg/1
  FyF1/1 -> mux/29
  FyJB/1 -> mux/131
  FrollHL22/1 -> mux/123
  demux/100 -> xRM/1
  demux/2 -> yg/1
  demux/105 -> rollRM/1
  demux/5 -> yawg/1
  demux/72 -> zPF/1
  demux/115 -> pitchHL1/1
  demux/3 -> zg/1
  FyawMD/1 -> mux/26
  FzJB/1 -> mux/132
  demux/110 -> yawTM/1
  FrollIM/1 -> mux/81
  FrollJB/1 -> mux/135
  demux/6 -> rollg/1
  demux/67 -> pitchBF/1
  FzHL23/1 -> mux/126
  demux/160 -> Terminator21/1
  FzHL3/1 -> mux/108
  FpitchHL22/1 -> mux/121
  FpitchHL21/1 -> mux/115
  demux/70 -> xPF/1
  FrollHL21/1 -> mux/117
  FyawHL22/1 -> mux/122
  FxJB/1 -> mux/130
  demux/85 -> pitchMN/1
  FxHL22/1 -> mux/118
  FxHL23/1 -> mux/124
  FpitchHL2/1 -> mux/103
  FyHL2/1 -> mux/101
  FxHL1/1 -> mux/94
  FpitchHL3/1 -> mux/109
  FyHL21/1 -> mux/113
  demux/65 -> yBF/1
  demux/116 -> yawHL1/1
  FyawHL2/1 -> mux/104
  FxTM/1 -> mux/88
  FyHL3/1 -> mux/107
  FxHL3/1 -> mux/106
  FyawTM/1 -> mux/92
  FyawF2/1 -> mux/38
  demux/258 -> Terminator113/1
  FzHL2/1 -> mux/102
  FpitchTM/1 -> mux/91
  FyawHL3/1 -> mux/110
  FyawHL21/1 -> mux/116
  FyawHL1/1 -> mux/98
  FrollHL2/1 -> mux/105
  demux/24 -> Terminator5/1
  FrollHL1/1 -> mux/99
  demux/133 -> pitchHL21/1
  demux/178 -> Terminator39/1
  FyawIRM/1 -> mux/74
  demux/166 -> Terminator27/1
  FxIRM/1 -> mux/70
  FpitchRM/1 -> mux/85
  FyawMNR/1 -> mux/62
  demux/257 -> Terminator112/1
  FrollMNR/1 -> mux/63
  FpitchHL23/1 -> mux/127
  FyMN/1 -> mux/65
  FxRM/1 -> mux/82
  demux/51 -> rollF1/1
  demux/7 -> xHLgnd/1
  FrollMN/1 -> mux/69
  FpitchIM/1 -> mux/79
  demux/27 -> Terminator8/1
  FxMN/1 -> mux/64
  FzHL22/1 -> mux/120
  FzMN/1 -> mux/66
  FyIRM/1 -> mux/71
  demux/14 -> yHLgnd2/1
  FzMNR/1 -> mux/60
  FzBF/1 -> mux/48
  FrollIRM/1 -> mux/75
  demux/11 -> yawHLgnd/1
  demux/45 -> rollMD/1
  FzF0/1 -> mux/20
  FxHL2/1 -> mux/100
  FyawPF/1 -> mux/56
  demux/10 -> pitchHLgnd/1
  demux/20 -> Terminator1/1
  FpitchPF/1 -> mux/55
  demux/1 -> xg/1
  FrollF1/1 -> mux/33
  FrollF3/1 -> mux/45
  FxHL21/1 -> mux/112
  FzPF/1 -> mux/54
  demux/93 -> rollIRM/1
  FpitchBF/1 -> mux/49
  FyawF3/1 -> mux/44
  FxBF/1 -> mux/46
  FyawF0/1 -> mux/21
  FpitchF3/1 -> mux/43
  demux/47 -> yF1/1
  demux/119 -> yHL2/1
  demux/59 -> yF3/1
  FpitchF2/1 -> mux/37
  FyF2/1 -> mux/35
  apitchHLgnd2/1 -> mux/16
  azHLgnd2/1 -> mux/15
  ayHLgnd2/1 -> mux/14
  FxF2/1 -> mux/34
  arollHLgnd/1 -> mux/12
  FrollPF/1 -> mux/57
  FpitchF1/1 -> mux/31
  axHLgnd/1 -> mux/7
  FzRM/1 -> mux/84
  FxIM/1 -> mux/76
  ayawHLgnd/1 -> mux/11
  demux/230 -> Terminator85/1
  azHLgnd/1 -> mux/9
  ayawg/1 -> mux/5
  azg/1 -> mux/3
  demux/209 -> Terminator70/1
  demux/172 -> Terminator33/1
  demux/259 -> Terminator114/1
  demux/208 -> Terminator69/1
  demux/182 -> Terminator43/1
  FyMD/1 -> mux/23
  demux/200 -> Terminator61/1
  demux/207 -> Terminator68/1
  demux/151 -> pitchJB/1
  demux/201 -> Terminator62/1
  mux/1 -> SAS State-Space/1
  demux/205 -> Terminator66/1
  demux/114 -> zHL1/1
  demux/25 -> Terminator6/1
  demux/197 -> Terminator58/1
  FyawJB/1 -> mux/134
  demux/212 -> Terminator73/1
  demux/214 -> Terminator75/1
  demux/23 -> Terminator4/1
  demux/88 -> xIRM/1
  FpitchHL1/1 -> mux/97
  FrollF2/1 -> mux/39
  demux/188 -> Terminator49/1
  demux/111 -> rollTM/1
  demux/192 -> Terminator53/1
  demux/84 -> zMN/1
  demux/148 -> xJB/1
  demux/179 -> Terminator40/1
  demux/154 -> vxF0/1
  demux/87 -> rollMN/1
  demux/185 -> Terminator46/1
  demux/147 -> rollHL23/1
  demux/167 -> Terminator28/1
  demux/186 -> Terminator47/1
  demux/143 -> yHL23/1
  apitchHLgnd/1 -> mux/10
  ayawHLgnd2/1 -> mux/17
  FzTM/1 -> mux/90
  ayHLgnd/1 -> mux/8
  demux/21 -> Terminator2/1
  FrollRM/1 -> mux/87
  demux/61 -> pitchF3/1
  demux/55 -> pitchF2/1
  demux/83 -> yMN/1
  demux/16 -> pitchHLgnd2/1
  demux/18 -> rollHLgnd2/1
  arollg/1 -> mux/6
  ayg/1 -> mux/2
  demux/98 -> yawIM/1
  FrollBF/1 -> mux/51
  demux/97 -> pitchIM/1
  demux/195 -> Terminator56/1
  FyawBF/1 -> mux/50
  axHLgnd2/1 -> mux/13
  demux/187 -> Terminator48/1
  demux/189 -> Terminator50/1
  demux/221 -> Terminator82/1
  demux/181 -> Terminator42/1
  FyHL22/1 -> mux/119
  demux/156 -> vyawF0/1
  FyIM/1 -> mux/77
  demux/245 -> Terminator100/1
  FyMNR/1 -> mux/59
  demux/170 -> Terminator31/1
  demux/169 -> Terminator30/1
  demux/229 -> Terminator84/1
  FpitchIRM/1 -> mux/73
  demux/194 -> Terminator55/1
  demux/157 -> Terminator18/1
  demux/17 -> yawHLgnd2/1
  demux/42 -> zMD/1
  demux/196 -> Terminator57/1
  demux/180 -> Terminator41/1
  demux/90 -> zIRM/1
  demux/69 -> rollBF/1
  demux/71 -> yPF/1
  demux/39 -> yawF0/1
  FyHL23/1 -> mux/125
  FpitchMN/1 -> mux/67
  FxF3/1 -> mux/40
  demux/76 -> xMNR/1
  demux/193 -> Terminator54/1
  demux/37 -> xF0/1
  FyawMN/1 -> mux/68
  demux/190 -> Terminator51/1
  demux/138 -> zHL22/1
  demux/9 -> zHLgnd/1
  demux/184 -> Terminator45/1
  demux/161 -> Terminator22/1
  demux/217 -> Terminator78/1
  FpitchJB/1 -> mux/133
  demux/141 -> rollHL22/1
  FyawHL23/1 -> mux/128
  demux/95 -> yIM/1
  demux/12 -> rollHLgnd/1
  FyTM/1 -> mux/89
  demux/29 -> Terminator10/1
  demux/30 -> Terminator11/1
  demux/36 -> Terminator12/1
  demux/35 -> Terminator13/1
  demux/34 -> Terminator14/1
  demux/33 -> Terminator15/1
  demux/32 -> Terminator16/1
  demux/31 -> Terminator17/1
